simulink model "Sunroof_Auto"  (R2020b)
settings: Solver=VariableStepAuto  StartTime=0.0  StopTime=40  MaxStep=0.1  RelTol=1e-3
undefined symbols (not defined in the file or in its folder): sigbuilder_block
settings Model: Creator=99003759  LastModifiedBy=99003759

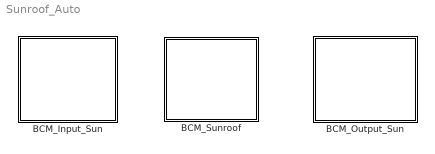
== system Sunroof_Auto ==
  BCM_Input_Sun : Subsystem
  BCM_Output_Sun : Subsystem
  BCM_Sunroof : Subsystem

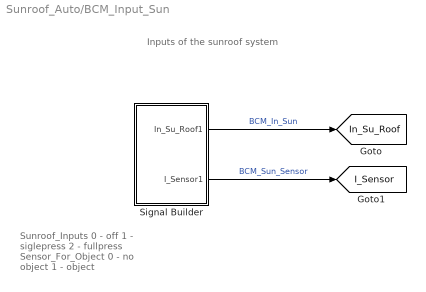
== system Sunroof_Auto/BCM_Input_Sun ==
  note: Inputs of the sunroof system
  note: Sunroof_Inputs
      | 0 - off
      | 1 - siglepress
      | 2 - fullpress
      | Sensor_For_Object
      | 0 - no object
      | 1 - object
  Signal Builder : Subsystem  Tag=STV Subsys  LoadFcn=sigbuilder_block('load');  StartFcn=sigbuilder_block('start');  StopFcn=sigbuilder_block('stop');  ClipboardFcn=sigbuilder_block('clipboard');  mask(Sigbuilder block){tuvar=[0:10]}
      mask help: Simulink:masks:SigbuilderBlock_MD
      mask init:
      | if ~strcmp(get_param(bdroot(gcbh),'SimulationStatus'),'stopped') tuvar = sigbuilder_block('maskInit'); end
      settings: CopyFcn=sigbuilder_block('copy');  DeleteFcn=sigbuilder_block('delete');  ModelCloseFcn=sigbuilder_block('modelClose');  PreSaveFcn=sigbuilder_block('preSave');  PauseFcn=sigbuilder_block('pause');  ContinueFcn=sigbuilder_block('continue');  NameChangeFcn=sigbuilder_block('namechange');  OpenFcn=sigbuilder_block('open',[408 139.5 550.5 359.25 ]);  CloseFcn=sigbuilder_block('close');
      mask Display: plot(0, 0, 100, 100,[2, 2, 32, 32, 2], [68, 8, 8, 68, 68],[32, 2], [38, 38], [32, 19, 2],[53, 60, 44], [32, 17, 17, 2],[16, 16, 31, 31]);txt = getActiveGroup(gcbh);text(2, 100, txt,'verticalAlignment', 'top');
  tag scope: I_Sensor=global, In_Su_Roof=global
  wires:
  Signal Builder/1(In_Su_Roof1) -> [In_Su_Roof]  "BCM_In_Sun"
  Signal Builder/2(I_Sensor1) -> [I_Sensor]  "BCM_Sun_Sensor"

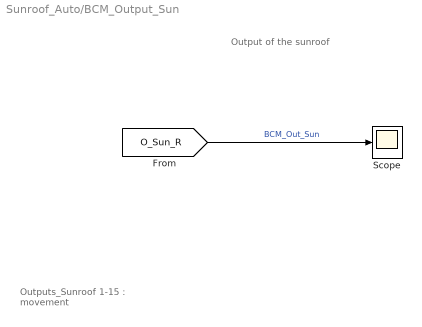
== system Sunroof_Auto/BCM_Output_Sun ==
  note: Output of the sunroof
  note: Outputs_Sunroof
      | 1-15 : movement
  Scope : Scope
  wires:
  [O_Sun_R] -> Scope/1  "BCM_Out_Sun"

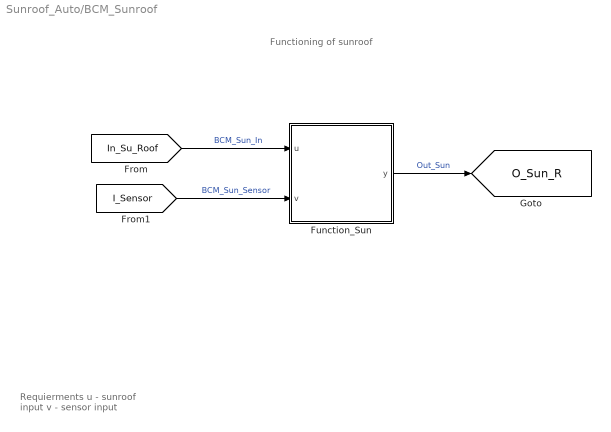
== system Sunroof_Auto/BCM_Sunroof ==
  note: Functioning of sunroof
  note: Requierments
      | u - sunroof input
      | v - sensor input
  Function_Sun : MATLAB Function  TreatAsAtomicUnit=on
  tag scope: O_Sun_R=global
  wires:
  Function_Sun/1(y) -> [O_Sun_R]  "Out_Sun"
  [I_Sensor] -> Function_Sun/2(v)  "BCM_Sun_Sensor"
  [In_Su_Roof] -> Function_Sun/1(u)  "BCM_Sun_In"

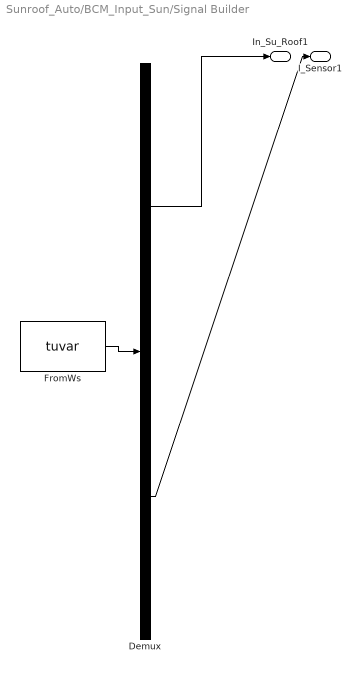
== system Sunroof_Auto/BCM_Input_Sun/Signal Builder ==
  Demux : Demux  Tag=STV Demux  Outputs=2
      settings: DisplayOption=none
  FromWs : FromWorkspace  Tag=STV FromWs  VariableName=tuvar
      SigBuilderData=|
      | common.afterFinalStr = 'Extrapolate'
      | common.sampleTime = 0
      | dataSet.timeRange = [0 10]
      | dataSet.name = 'Group 1'
      | sbobj.Groups.Name = 'Group 1'
      | sbobj.Groups.Signals(1).Name = 'In_Su_Roof1'
      | sbobj.Groups.Signals(1).XData = [0 1 2 3 4 5 6 7 8 9 10 11 12 13 14 15 16 17 18 19 20 21 22 23 24 25 26 27 28 29 30 31 32 33 34 35 36 37 38 39 40 41 42 43 44 45]
      | sbobj.Groups.Signals(1).YData = [0 1 2 3 3 2 1 1 0 1 2 3 3 2 1 0 1 1 2 3 3 2 1 0 1 2 3 3 2 2 1 1 0 0 1 1 2 2 3 3 2 2 1 1 1 0]
      | sbobj.Groups.Signals(2).Name = 'I_Sensor1'
      | sbobj.Groups.Signals(2).XData = [0 1 2 3 4 5 6 7 8 9 10 11 12 13 14 15 16 17 18 19 20 21 22 23 24 25 26 27 28 29 30 31 32 33 34 35 36 37 38 39 40 41 42 43 44 45]
      | sbobj.Groups.Signals(2).YData = [0 0 0 0 0 0 0 1 1 1 1 0 0 0 0 0 1 1 0 0 0 1 1 0 0 0 0 0 1 1 0 0 0 0 1 1 1 0 0 0 0 0 1 1 1 0]
  In_Su_Roof1 : Outport  Tag=STV Outport
  I_Sensor1 : Outport  Tag=STV Outport  Port=2
  wires:
  FromWs/1 -> Demux/1
  Demux/1 -> In_Su_Roof1/1
  Demux/2 -> I_Sensor1/1

== matlab function Sunroof_Auto/BCM_Sunroof/Function_Sun ==
  data: u input; y output; v input
function y = fcn(u,v)
if u == 1
    for i = 1:5
        y = u * i;
    end
elseif u == 2
    for i = 1:5
        y = u * i;
    end
elseif u == 3
    for i = 1:5
        y = u * i;
    end
else
    y = u;
end
if v == 1 && u ~= 0
   y = 15;
end
